simulink model "X5_PathTesting"  (R2024b)
settings: Solver=VariableStepAuto  StartTime=0.0  StopTime=20  RelTol=1e-3
libraries: Mako_Dynamics x3, dspinverses x2, g_block x1
(part 1 of 2)
settings Model: Creator=pinto  LastModifiedBy=pinto

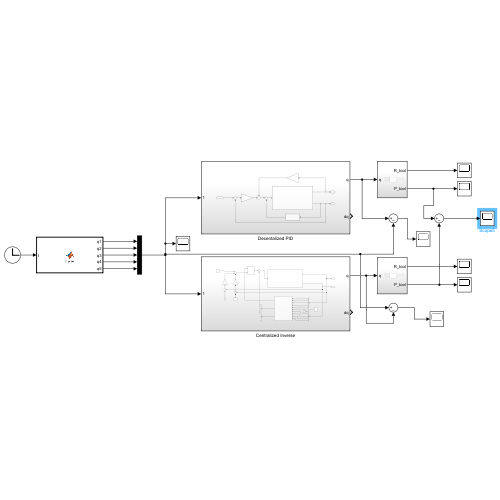
[thumbnail: Simulink's stored preview of the top-level diagram]
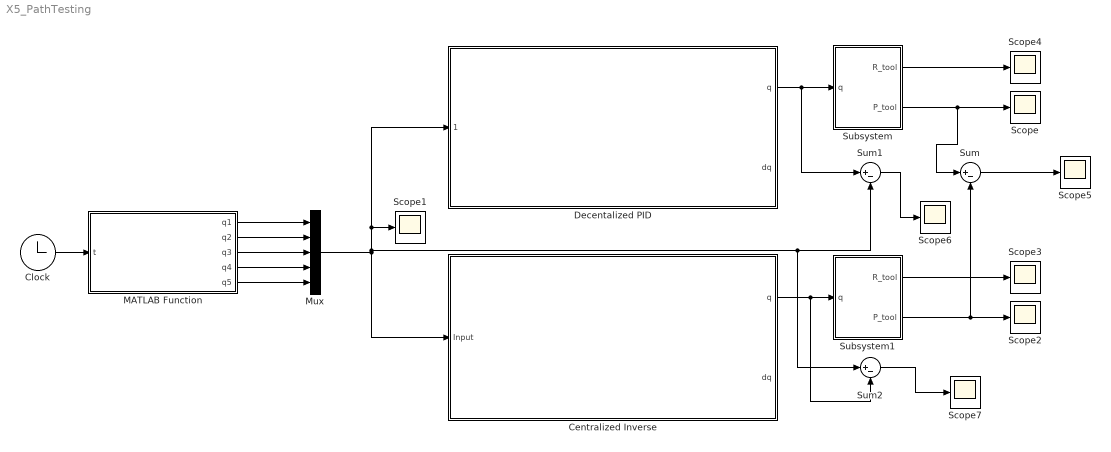
== system X5_PathTesting ==
  Centralized Inverse : Subsystem
  Clock : Clock
  Decentalized PID : Subsystem
  MATLAB Function : MATLAB Function  TreatAsAtomicUnit=on
  Mux : Mux  Inputs=5
  Scope{,1..7} (8 alike) : Scope
  Subsystem : Subsystem
  Subsystem1 : Subsystem
  Sum : Sum  Inputs=|+-
  Sum1 : Sum  Inputs=|+-
  Sum2 : Sum  Inputs=|+-
  wires:
  Clock/1 -> MATLAB Function/1(t)
  Decentalized PID/1(q) -> Sum1/1, Subsystem/1(q)
  Centralized Inverse/1(q) -> Sum2/2, Subsystem1/1(q)
  Subsystem/2(P_tool) -> Sum/1, Scope/1
  Subsystem1/2(P_tool) -> Sum/2, Scope2/1
  Subsystem1/1(R_tool) -> Scope3/1
  Subsystem/1(R_tool) -> Scope4/1
  Sum/1 -> Scope5/1
  MATLAB Function/2(q2) -> Mux/2
  Mux/1 -> Decentalized PID/1(1), Scope1/1, Sum2/1, Sum1/2, Centralized Inverse/1(Input)
  MATLAB Function/1(q1) -> Mux/1
  MATLAB Function/3(q3) -> Mux/3
  MATLAB Function/4(q4) -> Mux/4
  MATLAB Function/5(q5) -> Mux/5
  Sum1/1 -> Scope6/1
  Sum2/1 -> Scope7/1

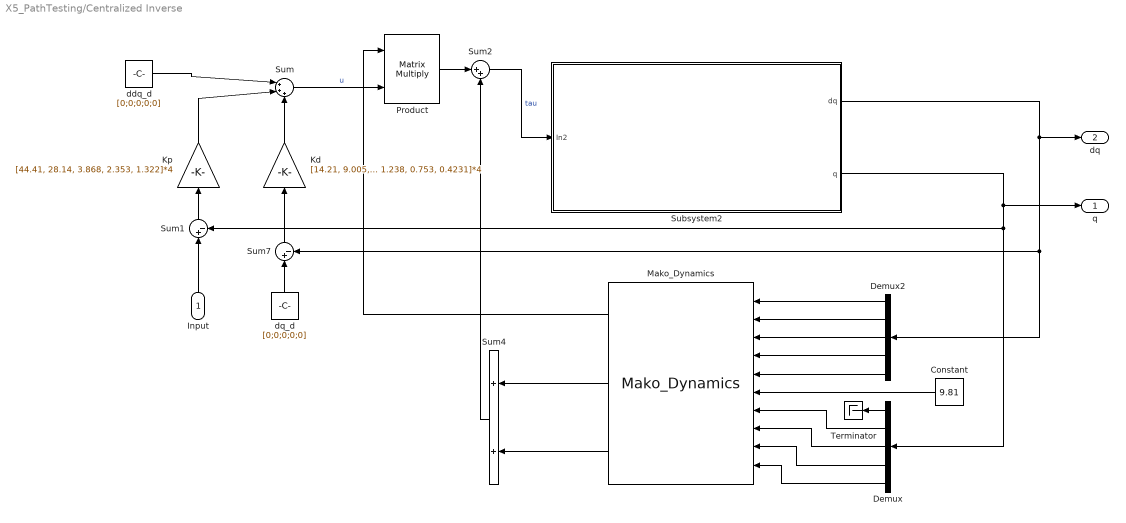
== system X5_PathTesting/Centralized Inverse ==
  Input : Inport
  Constant : Constant  Value=9.81
  Demux : Demux  Outputs=5
  Demux2 : Demux  Outputs=5
  Kd : Gain  Gain=[14.21, 9.005, 1.238, 0.753, 0.4231]*4
  Kp : Gain  Gain=[44.41, 28.14, 3.868, 2.353, 1.322]*4
  Mako_Dynamics : Mako_Dynamics/Mako_Dynamics  SystemSampleTime=-1  VariantActivationTime=update diagram  AllowFlexibleInterface=on  Latency=0  AutoFrameSizeCalculation=off
  Product : Product  Multiplication=Matrix(*)
  Subsystem2 : Subsystem
  Sum : Sum  Inputs=|+++
  Sum1 : Sum  Inputs=|+-
  Sum2 : Sum  Inputs=|++
  Sum4 : Sum
  Sum7 : Sum  Inputs=|+-
  Terminator : Terminator
  ddq_d : Constant  Value=[0;0;0;0;0]
  dq_d : Constant  Value=[0;0;0;0;0]
  q : Outport
  dq : Outport  Port=2
  wires:
  Demux/1 -> Terminator/1
  Demux2/1 -> Mako_Dynamics/1
  Kp/1 -> Sum/2
  ddq_d/1 -> Sum/1
  Product/1 -> Sum2/1
  Input/1 -> Sum1/1
  Subsystem2/2(q) -> Sum1/2, Demux/1, q/1
  Sum2/1 -> Subsystem2/1(In2)  "tau"
  Demux2/2 -> Mako_Dynamics/2
  Kd/1 -> Sum/3
  Sum1/1 -> Kp/1
  dq_d/1 -> Sum7/1
  Mako_Dynamics/1 -> Product/1
  Mako_Dynamics/3 -> Sum4/2
  Sum/1 -> Product/2  "u"
  Sum4/1 -> Sum2/2
  Demux2/3 -> Mako_Dynamics/3
  Subsystem2/1(dq) -> dq/1, Demux2/1, Sum7/2
  Sum7/1 -> Kd/1
  Demux2/5 -> Mako_Dynamics/5
  Demux2/4 -> Mako_Dynamics/4
  Mako_Dynamics/2 -> Sum4/1
  Demux/2 -> Mako_Dynamics/7
  Demux/3 -> Mako_Dynamics/8
  Demux/4 -> Mako_Dynamics/9
  Demux/5 -> Mako_Dynamics/10
  Constant/1 -> Mako_Dynamics/6

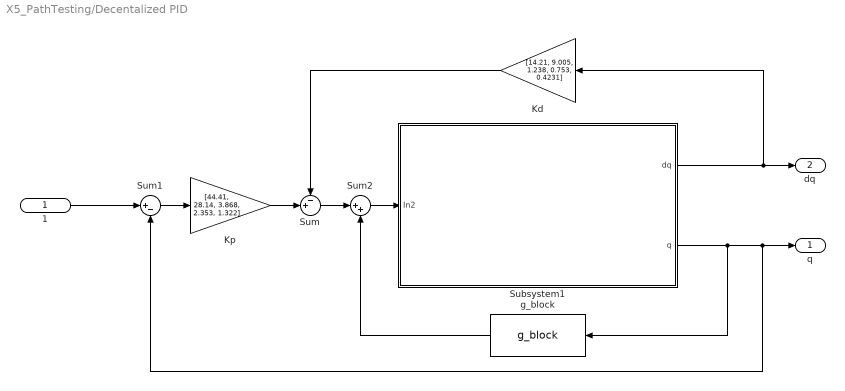
== system X5_PathTesting/Decentalized PID ==
  1 : Inport
  Kd : Gain  Gain=[14.21, 9.005, 1.238, 0.753, 0.4231]
  Kp : Gain  Gain=[44.41, 28.14, 3.868, 2.353, 1.322]
  Subsystem1 : Subsystem
  Sum : Sum  Inputs=-+|
  Sum1 : Sum  Inputs=|+-
  Sum2 : Sum  Inputs=|++
  g_block : g_block/g_block  SystemSampleTime=-1  VariantActivationTime=update diagram  AllowFlexibleInterface=on  Latency=0  AutoFrameSizeCalculation=off
  q : Outport
  dq : Outport  Port=2
  wires:
  Sum1/1 -> Kp/1
  1/1 -> Sum1/1
  Subsystem1/1(dq) -> dq/1, Kd/1
  Kd/1 -> Sum/1
  Sum2/1 -> Subsystem1/1(In2)
  Subsystem1/2(q) -> g_block/1, q/1, Sum1/2
  g_block/1 -> Sum2/2
  Kp/1 -> Sum/2
  Sum/1 -> Sum2/1

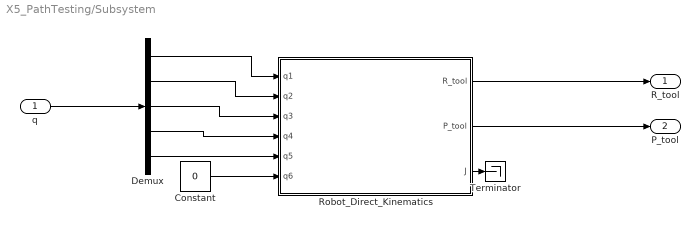
== system X5_PathTesting/Subsystem ==
  q : Inport
  Constant : Constant  Value=0
  Demux : Demux  Outputs=5
  Robot_Direct_Kinematics : MATLAB Function  TreatAsAtomicUnit=on
  Terminator : Terminator
  R_tool : Outport
  P_tool : Outport  Port=2
  wires:
  q/1 -> Demux/1
  Demux/1 -> Robot_Direct_Kinematics/1(q1)
  Demux/2 -> Robot_Direct_Kinematics/2(q2)
  Demux/3 -> Robot_Direct_Kinematics/3(q3)
  Demux/4 -> Robot_Direct_Kinematics/4(q4)
  Demux/5 -> Robot_Direct_Kinematics/5(q5)
  Constant/1 -> Robot_Direct_Kinematics/6(q6)
  Robot_Direct_Kinematics/1(R_tool) -> R_tool/1
  Robot_Direct_Kinematics/3(J) -> Terminator/1
  Robot_Direct_Kinematics/2(P_tool) -> P_tool/1

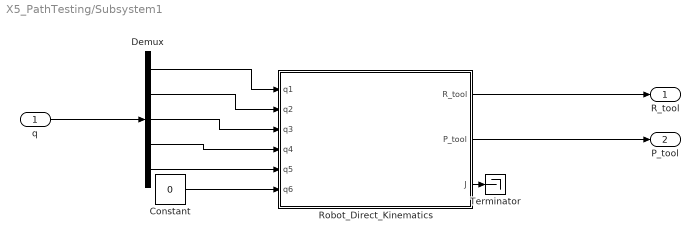
== system X5_PathTesting/Subsystem1 ==
  q : Inport
  Constant : Constant  Value=0
  Demux : Demux  Outputs=5
  Robot_Direct_Kinematics : MATLAB Function  TreatAsAtomicUnit=on
  Terminator : Terminator
  R_tool : Outport
  P_tool : Outport  Port=2
  wires:
  q/1 -> Demux/1
  Demux/1 -> Robot_Direct_Kinematics/1(q1)
  Demux/2 -> Robot_Direct_Kinematics/2(q2)
  Demux/3 -> Robot_Direct_Kinematics/3(q3)
  Demux/4 -> Robot_Direct_Kinematics/4(q4)
  Demux/5 -> Robot_Direct_Kinematics/5(q5)
  Constant/1 -> Robot_Direct_Kinematics/6(q6)
  Robot_Direct_Kinematics/1(R_tool) -> R_tool/1
  Robot_Direct_Kinematics/3(J) -> Terminator/1
  Robot_Direct_Kinematics/2(P_tool) -> P_tool/1

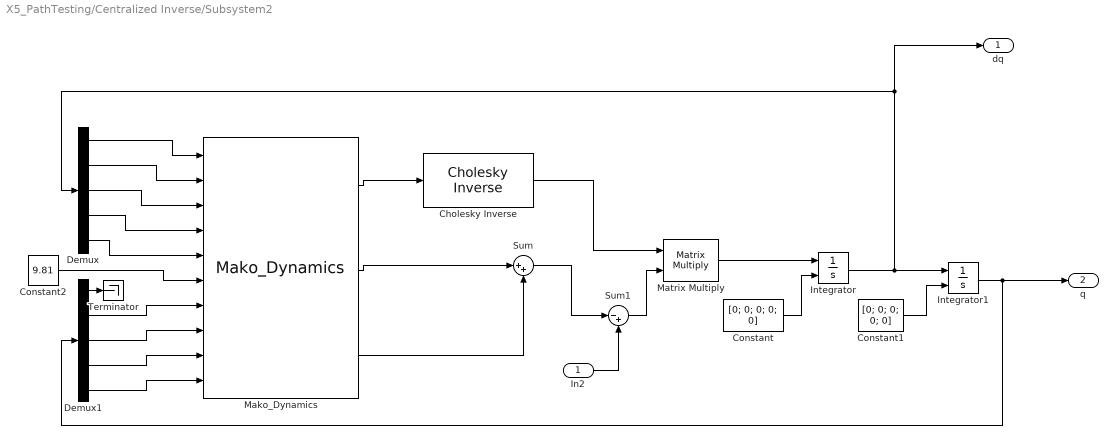
== system X5_PathTesting/Centralized Inverse/Subsystem2 ==
  In2 : Inport
  Cholesky Inverse : dspinverses/Cholesky Inverse  errmode=Warning
  Constant : Constant  Value=[0; 0; 0; 0; 0]
  Constant1 : Constant  Value=[0; 0; 0; 0; 0]
  Constant2 : Constant  Value=9.81
  Demux : Demux  Outputs=5
  Demux1 : Demux  Outputs=5
  Integrator : Integrator  InitialConditionSource=external  InitialCondition=[0.01, 0.01, 0.01]
  Integrator1 : Integrator  InitialConditionSource=external  InitialCondition=[0.01, 0.01, 0.01]
  Mako_Dynamics : Mako_Dynamics/Mako_Dynamics  SystemSampleTime=-1  VariantActivationTime=update diagram  AllowFlexibleInterface=on  Latency=0  AutoFrameSizeCalculation=off
  Matrix Multiply : Product  Multiplication=Matrix(*)
  Sum : Sum  Inputs=|++
  Sum1 : Sum  Inputs=|-+
  Terminator : Terminator
  dq : Outport
  q : Outport  Port=2
  wires:
  Sum/1 -> Sum1/1
  Demux/3 -> Mako_Dynamics/3
  Integrator/1 -> Integrator1/1, Demux/1, dq/1
  Matrix Multiply/1 -> Integrator/1
  Demux/4 -> Mako_Dynamics/4
  Demux/2 -> Mako_Dynamics/2
  Constant1/1 -> Integrator1/2
  Integrator1/1 -> q/1, Demux1/1
  Mako_Dynamics/1 -> Cholesky Inverse/1
  Cholesky Inverse/1 -> Matrix Multiply/1
  Constant/1 -> Integrator/2
  Sum1/1 -> Matrix Multiply/2
  Demux/1 -> Mako_Dynamics/1
  In2/1 -> Sum1/2
  Demux/5 -> Mako_Dynamics/5
  Mako_Dynamics/2 -> Sum/1
  Mako_Dynamics/3 -> Sum/2
  Demux1/1 -> Terminator/1
  Constant2/1 -> Mako_Dynamics/6
  Demux1/2 -> Mako_Dynamics/7
  Demux1/3 -> Mako_Dynamics/8
  Demux1/4 -> Mako_Dynamics/9
  Demux1/5 -> Mako_Dynamics/10

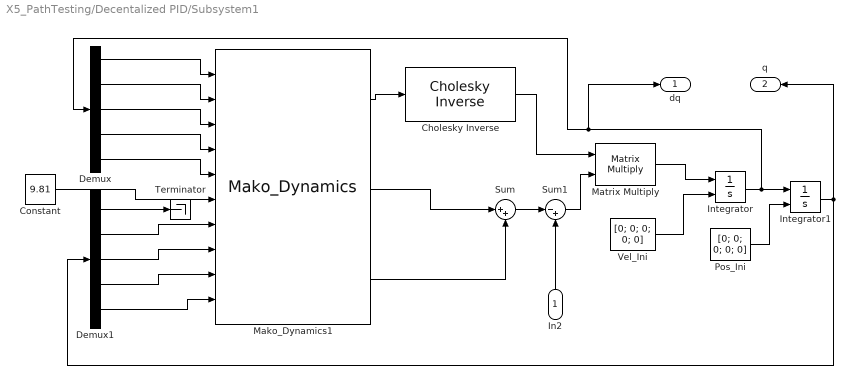
== system X5_PathTesting/Decentalized PID/Subsystem1 ==
  In2 : Inport
  Cholesky Inverse : dspinverses/Cholesky Inverse  errmode=Warning
  Constant : Constant  Value=9.81
  Demux : Demux  Outputs=5
  Demux1 : Demux  Outputs=5
  Integrator : Integrator  InitialConditionSource=external  InitialCondition=[0.01, 0.01, 0.01]
  Integrator1 : Integrator  InitialConditionSource=external  InitialCondition=[0.01, 0.01, 0.01]
  Mako_Dynamics1 : Mako_Dynamics/Mako_Dynamics  SystemSampleTime=-1  VariantActivationTime=update diagram  AllowFlexibleInterface=on  Latency=0  AutoFrameSizeCalculation=off
  Matrix Multiply : Product  Multiplication=Matrix(*)
  Pos_Ini : Constant  Value=[0; 0; 0; 0; 0]
  Sum : Sum  Inputs=|++
  Sum1 : Sum  Inputs=|-+
  Terminator : Terminator
  Vel_Ini : Constant  Value=[0; 0; 0; 0; 0]
  dq : Outport
  q : Outport  Port=2
  wires:
  Sum/1 -> Sum1/1
  Mako_Dynamics1/3 -> Sum/2
  Demux/3 -> Mako_Dynamics1/3
  Integrator/1 -> Integrator1/1, Demux/1, dq/1
  Matrix Multiply/1 -> Integrator/1
  Demux/4 -> Mako_Dynamics1/4
  Demux/2 -> Mako_Dynamics1/2
  Pos_Ini/1 -> Integrator1/2
  Integrator1/1 -> q/1, Demux1/1
  Mako_Dynamics1/1 -> Cholesky Inverse/1
  Cholesky Inverse/1 -> Matrix Multiply/1
  Vel_Ini/1 -> Integrator/2
  Sum1/1 -> Matrix Multiply/2
  Demux/1 -> Mako_Dynamics1/1
  In2/1 -> Sum1/2
  Mako_Dynamics1/2 -> Sum/1
  Demux/5 -> Mako_Dynamics1/5
  Demux1/1 -> Terminator/1
  Constant/1 -> Mako_Dynamics1/6
  Demux1/2 -> Mako_Dynamics1/7
  Demux1/3 -> Mako_Dynamics1/8
  Demux1/4 -> Mako_Dynamics1/9
  Demux1/5 -> Mako_Dynamics1/10

== matlab function X5_PathTesting/MATLAB Function ==
  data: t input; q1 output; q2 output; q3 output; q4 output; q5 output
function [q1,q2,q3,q4,q5] = Path(t)
    T = 20;
    t = min(max(t,0),T);
    s = 4*(t/T)*(1 - t/T);

    q_start = [0; 0; 0; 0; 0];
    q_peak  = [-0.4; -0.3; -0.2; 0.3; 0.3];
    q       = q_start + s*(q_peak - q_start);

    q1 = q(1);
    q2 = q(2);
    q3 = q(3);
    q4 = q(4);
    q5 = q(5);
end

== matlab function X5_PathTesting/Subsystem/Robot_Direct_Kinematics ==
  data: q1 input; R_tool output; q2 input; q3 input; q4 input; q5 input; q6 input; P_tool output; J output
function [R_tool,P_tool,J] = Robot_Direct_Kinematics(q1,q2,q3,q4,q5,q6)
%#codegen

%    This function was generated by the Symbolic Math Toolbox version 24.2.
%    24-May-2025 22:37:09

% q1 = complex(q1);  % if required to enforce complex operations
% q2 = complex(q2);  % if required to enforce complex operations
% q3 = complex(q3);  % if required to enforce complex operations
% q4 = complex(q4);  % if required to enforce complex operations
% q5 = complex(q5);  % if required to enforce complex operations
% q6 = complex(q6);  % if required to enforce complex operations
et1 = cos(q5).*sin(q1).*sin(q3).*sqrt(sqrt(2.0)+2.0).*(-1.0./2.0)-(cos(q1).*cos(q2).*sin(q4).*sin(q6).*sqrt(-sqrt(2.0)+2.0))./2.0-(cos(q3).*cos(q4).*sin(q1).*sin(q6).*sqrt(-sqrt(2.0)+2.0))./2.0-(cos(q6).*sin(q1).*sin(q3).*sin(q5).*sqrt(-sqrt(2.0)+2.0))./2.0-(cos(q1).*cos(q3).*cos(q5).*sin(q2).*sqrt(sqrt(2.0)+2.0))./2.0-(cos(q1).*cos(q2).*cos(q4).*sin(q5).*sqrt(sqrt(2.0)+2.0))./2.0+(cos(q3).*sin(q1).*sin(q4).*sin(q5).*sqrt(sqrt(2.0)+2.0))./2.0;
et2 = (cos(q1).*cos(q2).*cos(q4).*cos(q5).*cos(q6).*sqrt(-sqrt(2.0)+2.0))./2.0-(cos(q1).*cos(q3).*cos(q6).*sin(q2).*sin(q5).*sqrt(-sqrt(2.0)+2.0))./2.0-(cos(q3).*cos(q5).*cos(q6).*sin(q1).*sin(q4).*sqrt(-sqrt(2.0)+2.0))./2.0+(cos(q1).*cos(q4).*sin(q2).*sin(q3).*sin(q6).*sqrt(-sqrt(2.0)+2.0))./2.0-(cos(q1).*sin(q2).*sin(q3).*sin(q4).*sin(q5).*sqrt(sqrt(2.0)+2.0))./2.0+(cos(q1).*cos(q5).*cos(q6).*sin(q2).*sin(q3).*sin(q4).*sqrt(-sqrt(2.0)+2.0))./2.0;
et3 = cos(q1).*cos(q5).*sin(q3).*sqrt(sqrt(2.0)+2.0).*(-1.0./2.0)-(cos(q1).*cos(q3).*cos(q4).*sin(q6).*sqrt(-sqrt(2.0)+2.0))./2.0-(cos(q1).*cos(q6).*sin(q3).*sin(q5).*sqrt(-sqrt(2.0)+2.0))./2.0+(cos(q2).*sin(q1).*sin(q4).*sin(q6).*sqrt(-sqrt(2.0)+2.0))./2.0+(cos(q3).*cos(q5).*sin(q1).*sin(q2).*sqrt(sqrt(2.0)+2.0))./2.0+(cos(q2).*cos(q4).*sin(q1).*sin(q5).*sqrt(sqrt(2.0)+2.0))./2.0+(cos(q1).*cos(q3).*sin(q4).*sin(q5).*sqrt(sqrt(2.0)+2.0))./2.0-(cos(q2).*cos(q4).*cos(q5).*cos(q6).*sin(q1).*sqrt(-sqrt(2.0)+2.0))./2.0;
et4 = cos(q1).*cos(q3).*cos(q5).*cos(q6).*sin(q4).*sqrt(-sqrt(2.0)+2.0).*(-1.0./2.0)+(cos(q3).*cos(q6).*sin(q1).*sin(q2).*sin(q5).*sqrt(-sqrt(2.0)+2.0))./2.0-(cos(q4).*sin(q1).*sin(q2).*sin(q3).*sin(q6).*sqrt(-sqrt(2.0)+2.0))./2.0+(sin(q1).*sin(q2).*sin(q3).*sin(q4).*sin(q5).*sqrt(sqrt(2.0)+2.0))./2.0-(cos(q5).*cos(q6).*sin(q1).*sin(q2).*sin(q3).*sin(q4).*sqrt(-sqrt(2.0)+2.0))./2.0;
et5 = cos(q5).*sin(q1).*sin(q3).*sqrt(-sqrt(2.0)+2.0).*(-1.0./2.0)-(cos(q1).*cos(q3).*cos(q5).*sin(q2).*sqrt(-sqrt(2.0)+2.0))./2.0-(cos(q1).*cos(q2).*cos(q4).*sin(q5).*sqrt(-sqrt(2.0)+2.0))./2.0+(cos(q3).*sin(q1).*sin(q4).*sin(q5).*sqrt(-sqrt(2.0)+2.0))./2.0+(cos(q1).*cos(q2).*sin(q4).*sin(q6).*sqrt(sqrt(2.0)+2.0))./2.0+(cos(q3).*cos(q4).*sin(q1).*sin(q6).*sqrt(sqrt(2.0)+2.0))./2.0+(cos(q6).*sin(q1).*sin(q3).*sin(q5).*sqrt(sqrt(2.0)+2.0))./2.0;
et6 = cos(q1).*sin(q2).*sin(q3).*sin(q4).*sin(q5).*sqrt(-sqrt(2.0)+2.0).*(-1.0./2.0)-(cos(q1).*cos(q2).*cos(q4).*cos(q5).*cos(q6).*sqrt(sqrt(2.0)+2.0))./2.0+(cos(q1).*cos(q3).*cos(q6).*sin(q2).*sin(q5).*sqrt(sqrt(2.0)+2.0))./2.0+(cos(q3).*cos(q5).*cos(q6).*sin(q1).*sin(q4).*sqrt(sqrt(2.0)+2.0))./2.0-(cos(q1).*cos(q4).*sin(q2).*sin(q3).*sin(q6).*sqrt(sqrt(2.0)+2.0))./2.0-(cos(q1).*cos(q5).*cos(q6).*sin(q2).*sin(q3).*sin(q4).*sqrt(sqrt(2.0)+2.0))./2.0;
et7 = cos(q1).*cos(q5).*sin(q3).*sqrt(-sqrt(2.0)+2.0).*(-1.0./2.0)+(cos(q3).*cos(q5).*sin(q1).*sin(q2).*sqrt(-sqrt(2.0)+2.0))./2.0+(cos(q2).*cos(q4).*sin(q1).*sin(q5).*sqrt(-sqrt(2.0)+2.0))./2.0+(cos(q1).*cos(q3).*sin(q4).*sin(q5).*sqrt(-sqrt(2.0)+2.0))./2.0+(cos(q1).*cos(q3).*cos(q4).*sin(q6).*sqrt(sqrt(2.0)+2.0))./2.0+(cos(q1).*cos(q6).*sin(q3).*sin(q5).*sqrt(sqrt(2.0)+2.0))./2.0-(cos(q2).*sin(q1).*sin(q4).*sin(q6).*sqrt(sqrt(2.0)+2.0))./2.0;
et8 = (sin(q1).*sin(q2).*sin(q3).*sin(q4).*sin(q5).*sqrt(-sqrt(2.0)+2.0))./2.0+(cos(q2).*cos(q4).*cos(q5).*cos(q6).*sin(q1).*sqrt(sqrt(2.0)+2.0))./2.0+(cos(q1).*cos(q3).*cos(q5).*cos(q6).*sin(q4).*sqrt(sqrt(2.0)+2.0))./2.0-(cos(q3).*cos(q6).*sin(q1).*sin(q2).*sin(q5).*sqrt(sqrt(2.0)+2.0))./2.0+(cos(q4).*sin(q1).*sin(q2).*sin(q3).*sin(q6).*sqrt(sqrt(2.0)+2.0))./2.0+(cos(q5).*cos(q6).*sin(q1).*sin(q2).*sin(q3).*sin(q4).*sqrt(sqrt(2.0)+2.0))./2.0;
mt1 = [cos(q1).*cos(q3).*cos(q4).*cos(q6)-cos(q2).*cos(q6).*sin(q1).*sin(q4)-cos(q1).*sin(q3).*sin(q5).*sin(q6)-cos(q2).*cos(q4).*cos(q5).*sin(q1).*sin(q6)-cos(q1).*cos(q3).*cos(q5).*sin(q4).*sin(q6)+cos(q4).*cos(q6).*sin(q1).*sin(q2).*sin(q3)+cos(q3).*sin(q1).*sin(q2).*sin(q5).*sin(q6)-cos(q5).*sin(q1).*sin(q2).*sin(q3).*sin(q4).*sin(q6),cos(q1).*cos(q2).*cos(q6).*sin(q4)+cos(q3).*cos(q4).*cos(q6).*sin(q1)-sin(q1).*sin(q3).*sin(q5).*sin(q6)+cos(q1).*cos(q2).*cos(q4).*cos(q5).*sin(q6)-cos(q1).*cos(q4).*cos(q6).*sin(q2).*sin(q3)-cos(q1).*cos(q3).*sin(q2).*sin(q5).*sin(q6)-cos(q3).*cos(q5).*sin(q1).*sin(q4).*sin(q6)+cos(q1).*cos(q5).*sin(q2).*sin(q3).*sin(q4).*sin(q6)];
mt2 = [cos(q6).*sin(q2).*sin(q4)+cos(q2).*cos(q4).*cos(q6).*sin(q3)+cos(q2).*cos(q3).*sin(q5).*sin(q6)+cos(q4).*cos(q5).*sin(q2).*sin(q6)-cos(q2).*cos(q5).*sin(q3).*sin(q4).*sin(q6),et3+et4,et1+et2];
mt3 = [cos(q4).*sin(q2).*sin(q5).*sqrt(sqrt(2.0)+2.0).*(-1.0./2.0)-(sin(q2).*sin(q4).*sin(q6).*sqrt(-sqrt(2.0)+2.0))./2.0+(cos(q2).*cos(q3).*cos(q5).*sqrt(sqrt(2.0)+2.0))./2.0+(cos(q2).*cos(q3).*cos(q6).*sin(q5).*sqrt(-sqrt(2.0)+2.0))./2.0+(cos(q4).*cos(q5).*cos(q6).*sin(q2).*sqrt(-sqrt(2.0)+2.0))./2.0-(cos(q2).*cos(q4).*sin(q3).*sin(q6).*sqrt(-sqrt(2.0)+2.0))./2.0+(cos(q2).*sin(q3).*sin(q4).*sin(q5).*sqrt(sqrt(2.0)+2.0))./2.0-(cos(q2).*cos(q5).*cos(q6).*sin(q3).*sin(q4).*sqrt(-sqrt(2.0)+2.0))./2.0];
mt4 = [et7+et8,et5+et6,(sin(q2).*sin(q4).*sin(q6).*sqrt(sqrt(2.0)+2.0))./2.0+(cos(q2).*cos(q3).*cos(q5).*sqrt(-sqrt(2.0)+2.0))./2.0-(cos(q4).*sin(q2).*sin(q5).*sqrt(-sqrt(2.0)+2.0))./2.0+(cos(q2).*sin(q3).*sin(q4).*sin(q5).*sqrt(-sqrt(2.0)+2.0))./2.0-(cos(q2).*cos(q3).*cos(q6).*sin(q5).*sqrt(sqrt(2.0)+2.0))./2.0-(cos(q4).*cos(q5).*cos(q6).*sin(q2).*sqrt(sqrt(2.0)+2.0))./2.0+(cos(q2).*cos(q4).*sin(q3).*sin(q6).*sqrt(sqrt(2.0)+2.0))./2.0+(cos(q2).*cos(q5).*cos(q6).*sin(q3).*sin(q4).*sqrt(sqrt(2.0)+2.0))./2.0];
R_tool = reshape([mt1,mt2,mt3,mt4],3,3);
if nargout > 1
    et9 = sin(q2).*(2.0./5.0)+(cos(q4).*sin(q2))./1.0e+1+(sin(q2).*sin(q4))./2.0-(cos(q2).*cos(q3).*cos(q5))./1.0e+1+(cos(q2).*cos(q4).*sin(q3))./2.0-(cos(q2).*sin(q3).*sin(q4))./1.0e+1+(cos(q4).*sin(q2).*sin(q5))./1.0e+1+sin(q2).*sin(q4).*sin(q6).*sqrt(sqrt(2.0)+2.0).*(3.0./4.0e+1)+cos(q2).*cos(q3).*cos(q5).*sqrt(-sqrt(2.0)+2.0).*(3.0./4.0e+1)-cos(q4).*sin(q2).*sin(q5).*sqrt(-sqrt(2.0)+2.0).*(3.0./4.0e+1)-(cos(q2).*sin(q3).*sin(q4).*sin(q5))./1.0e+1+cos(q2).*sin(q3).*sin(q4).*sin(q5).*sqrt(-sqrt(2.0)+2.0).*(3.0./4.0e+1);
    et10 = cos(q2).*cos(q3).*cos(q6).*sin(q5).*sqrt(sqrt(2.0)+2.0).*(-3.0./4.0e+1)-cos(q4).*cos(q5).*cos(q6).*sin(q2).*sqrt(sqrt(2.0)+2.0).*(3.0./4.0e+1)+cos(q2).*cos(q4).*sin(q3).*sin(q6).*sqrt(sqrt(2.0)+2.0).*(3.0./4.0e+1)+cos(q2).*cos(q5).*cos(q6).*sin(q3).*sin(q4).*sqrt(sqrt(2.0)+2.0).*(3.0./4.0e+1);
    et11 = cos(q1).*cos(q2).*(2.0./5.0)+(cos(q1).*cos(q2).*cos(q4))./1.0e+1+(cos(q1).*cos(q2).*sin(q4))./2.0+(cos(q3).*cos(q4).*sin(q1))./2.0-(cos(q3).*sin(q1).*sin(q4))./1.0e+1+(cos(q5).*sin(q1).*sin(q3))./1.0e+1-cos(q5).*sin(q1).*sin(q3).*sqrt(-sqrt(2.0)+2.0).*(3.0./4.0e+1)+(cos(q1).*cos(q3).*cos(q5).*sin(q2))./1.0e+1+(cos(q1).*cos(q2).*cos(q4).*sin(q5))./1.0e+1-(cos(q1).*cos(q4).*sin(q2).*sin(q3))./2.0+(cos(q1).*sin(q2).*sin(q3).*sin(q4))./1.0e+1-(cos(q3).*sin(q1).*sin(q4).*sin(q5))./1.0e+1-cos(q1).*cos(q3).*cos(q5).*sin(q2).*sqrt(-sqrt(2.0)+2.0).*(3.0./4.0e+1);
    et12 = cos(q1).*cos(q2).*cos(q4).*sin(q5).*sqrt(-sqrt(2.0)+2.0).*(-3.0./4.0e+1)+cos(q3).*sin(q1).*sin(q4).*sin(q5).*sqrt(-sqrt(2.0)+2.0).*(3.0./4.0e+1)+(cos(q1).*sin(q2).*sin(q3).*sin(q4).*sin(q5))./1.0e+1+cos(q1).*cos(q2).*sin(q4).*sin(q6).*sqrt(sqrt(2.0)+2.0).*(3.0./4.0e+1)+cos(q3).*cos(q4).*sin(q1).*sin(q6).*sqrt(sqrt(2.0)+2.0).*(3.0./4.0e+1)+cos(q6).*sin(q1).*sin(q3).*sin(q5).*sqrt(sqrt(2.0)+2.0).*(3.0./4.0e+1)-cos(q1).*sin(q2).*sin(q3).*sin(q4).*sin(q5).*sqrt(-sqrt(2.0)+2.0).*(3.0./4.0e+1)-cos(q1).*cos(q2).*cos(q4).*cos(q5).*cos(q6).*sqrt(sqrt(2.0)+2.0).*(3.0./4.0e+1);
    et13 = cos(q1).*cos(q3).*cos(q6).*sin(q2).*sin(q5).*sqrt(sqrt(2.0)+2.0).*(3.0./4.0e+1)+cos(q3).*cos(q5).*cos(q6).*sin(q1).*sin(q4).*sqrt(sqrt(2.0)+2.0).*(3.0./4.0e+1)-cos(q1).*cos(q4).*sin(q2).*sin(q3).*sin(q6).*sqrt(sqrt(2.0)+2.0).*(3.0./4.0e+1)-cos(q1).*cos(q5).*cos(q6).*sin(q2).*sin(q3).*sin(q4).*sqrt(sqrt(2.0)+2.0).*(3.0./4.0e+1);
    et14 = cos(q2).*sin(q1).*(-2.0./5.0)+(cos(q1).*cos(q3).*cos(q4))./2.0-(cos(q2).*cos(q4).*sin(q1))./1.0e+1-(cos(q1).*cos(q3).*sin(q4))./1.0e+1+(cos(q1).*cos(q5).*sin(q3))./1.0e+1-(cos(q2).*sin(q1).*sin(q4))./2.0-cos(q1).*cos(q5).*sin(q3).*sqrt(-sqrt(2.0)+2.0).*(3.0./4.0e+1)-(cos(q3).*cos(q5).*sin(q1).*sin(q2))./1.0e+1-(cos(q2).*cos(q4).*sin(q1).*sin(q5))./1.0e+1-(cos(q1).*cos(q3).*sin(q4).*sin(q5))./1.0e+1+(cos(q4).*sin(q1).*sin(q2).*sin(q3))./2.0-(sin(q1).*sin(q2).*sin(q3).*sin(q4))./1.0e+1+cos(q3).*cos(q5).*sin(q1).*sin(q2).*sqrt(-sqrt(2.0)+2.0).*(3.0./4.0e+1);
    et15 = cos(q2).*cos(q4).*sin(q1).*sin(q5).*sqrt(-sqrt(2.0)+2.0).*(3.0./4.0e+1)+cos(q1).*cos(q3).*sin(q4).*sin(q5).*sqrt(-sqrt(2.0)+2.0).*(3.0./4.0e+1)-(sin(q1).*sin(q2).*sin(q3).*sin(q4).*sin(q5))./1.0e+1+cos(q1).*cos(q3).*cos(q4).*sin(q6).*sqrt(sqrt(2.0)+2.0).*(3.0./4.0e+1)+cos(q1).*cos(q6).*sin(q3).*sin(q5).*sqrt(sqrt(2.0)+2.0).*(3.0./4.0e+1)-cos(q2).*sin(q1).*sin(q4).*sin(q6).*sqrt(sqrt(2.0)+2.0).*(3.0./4.0e+1)+sin(q1).*sin(q2).*sin(q3).*sin(q4).*sin(q5).*sqrt(-sqrt(2.0)+2.0).*(3.0./4.0e+1)+cos(q2).*cos(q4).*cos(q5).*cos(q6).*sin(q1).*sqrt(sqrt(2.0)+2.0).*(3.0./4.0e+1);
    et16 = cos(q1).*cos(q3).*cos(q5).*cos(q6).*sin(q4).*sqrt(sqrt(2.0)+2.0).*(3.0./4.0e+1)-cos(q3).*cos(q6).*sin(q1).*sin(q2).*sin(q5).*sqrt(sqrt(2.0)+2.0).*(3.0./4.0e+1)+cos(q4).*sin(q1).*sin(q2).*sin(q3).*sin(q6).*sqrt(sqrt(2.0)+2.0).*(3.0./4.0e+1)+cos(q5).*cos(q6).*sin(q1).*sin(q2).*sin(q3).*sin(q4).*sqrt(sqrt(2.0)+2.0).*(3.0./4.0e+1);
    P_tool = [et14+et15+et16;et11+et12+et13;et9+et10];
end
if nargout > 2
    et17 = cos(q2).*sin(q1).*(-2.0./5.0)+(cos(q1).*cos(q3).*cos(q4))./2.0-(cos(q2).*cos(q4).*sin(q1))./1.0e+1-(cos(q1).*cos(q3).*sin(q4))./1.0e+1+(cos(q1).*cos(q5).*sin(q3))./1.0e+1-(cos(q2).*sin(q1).*sin(q4))./2.0-cos(q1).*cos(q5).*sin(q3).*sqrt(-sqrt(2.0)+2.0).*(3.0./4.0e+1)-(cos(q3).*cos(q5).*sin(q1).*sin(q2))./1.0e+1-(cos(q2).*cos(q4).*sin(q1).*sin(q5))./1.0e+1-(cos(q1).*cos(q3).*sin(q4).*sin(q5))./1.0e+1+(cos(q4).*sin(q1).*sin(q2).*sin(q3))./2.0-(sin(q1).*sin(q2).*sin(q3).*sin(q4))./1.0e+1+cos(q3).*cos(q5).*sin(q1).*sin(q2).*sqrt(-sqrt(2.0)+2.0).*(3.0./4.0e+1);
    et18 = cos(q2).*cos(q4).*sin(q1).*sin(q5).*sqrt(-sqrt(2.0)+2.0).*(3.0./4.0e+1)+cos(q1).*cos(q3).*sin(q4).*sin(q5).*sqrt(-sqrt(2.0)+2.0).*(3.0./4.0e+1)-(sin(q1).*sin(q2).*sin(q3).*sin(q4).*sin(q5))./1.0e+1+cos(q1).*cos(q3).*cos(q4).*sin(q6).*sqrt(sqrt(2.0)+2.0).*(3.0./4.0e+1)+cos(q1).*cos(q6).*sin(q3).*sin(q5).*sqrt(sqrt(2.0)+2.0).*(3.0./4.0e+1)-cos(q2).*sin(q1).*sin(q4).*sin(q6).*sqrt(sqrt(2.0)+2.0).*(3.0./4.0e+1)+sin(q1).*sin(q2).*sin(q3).*sin(q4).*sin(q5).*sqrt(-sqrt(2.0)+2.0).*(3.0./4.0e+1)+cos(q2).*cos(q4).*cos(q5).*cos(q6).*sin(q1).*sqrt(sqrt(2.0)+2.0).*(3.0./4.0e+1);
    et19 = cos(q1).*cos(q3).*cos(q5).*cos(q6).*sin(q4).*sqrt(sqrt(2.0)+2.0).*(3.0./4.0e+1)-cos(q3).*cos(q6).*sin(q1).*sin(q2).*sin(q5).*sqrt(sqrt(2.0)+2.0).*(3.0./4.0e+1)+cos(q4).*sin(q1).*sin(q2).*sin(q3).*sin(q6).*sqrt(sqrt(2.0)+2.0).*(3.0./4.0e+1)+cos(q5).*cos(q6).*sin(q1).*sin(q2).*sin(q3).*sin(q4).*sqrt(sqrt(2.0)+2.0).*(3.0./4.0e+1);
    et20 = cos(q1).*cos(q2).*(-2.0./5.0)-(cos(q1).*cos(q2).*cos(q4))./1.0e+1-(cos(q1).*cos(q2).*sin(q4))./2.0-(cos(q3).*cos(q4).*sin(q1))./2.0+(cos(q3).*sin(q1).*sin(q4))./1.0e+1-(cos(q5).*sin(q1).*sin(q3))./1.0e+1+cos(q5).*sin(q1).*sin(q3).*sqrt(-sqrt(2.0)+2.0).*(3.0./4.0e+1)-(cos(q1).*cos(q3).*cos(q5).*sin(q2))./1.0e+1-(cos(q1).*cos(q2).*cos(q4).*sin(q5))./1.0e+1+(cos(q1).*cos(q4).*sin(q2).*sin(q3))./2.0-(cos(q1).*sin(q2).*sin(q3).*sin(q4))./1.0e+1+(cos(q3).*sin(q1).*sin(q4).*sin(q5))./1.0e+1+cos(q1).*cos(q3).*cos(q5).*sin(q2).*sqrt(-sqrt(2.0)+2.0).*(3.0./4.0e+1);
    et21 = cos(q1).*cos(q2).*cos(q4).*sin(q5).*sqrt(-sqrt(2.0)+2.0).*(3.0./4.0e+1)-cos(q3).*sin(q1).*sin(q4).*sin(q5).*sqrt(-sqrt(2.0)+2.0).*(3.0./4.0e+1)-(cos(q1).*sin(q2).*sin(q3).*sin(q4).*sin(q5))./1.0e+1-cos(q1).*cos(q2).*sin(q4).*sin(q6).*sqrt(sqrt(2.0)+2.0).*(3.0./4.0e+1)-cos(q3).*cos(q4).*sin(q1).*sin(q6).*sqrt(sqrt(2.0)+2.0).*(3.0./4.0e+1)-cos(q6).*sin(q1).*sin(q3).*sin(q5).*sqrt(sqrt(2.0)+2.0).*(3.0./4.0e+1)+cos(q1).*sin(q2).*sin(q3).*sin(q4).*sin(q5).*sqrt(-sqrt(2.0)+2.0).*(3.0./4.0e+1);
    et22 = cos(q1).*cos(q2).*cos(q4).*cos(q5).*cos(q6).*sqrt(sqrt(2.0)+2.0).*(3.0./4.0e+1)-cos(q1).*cos(q3).*cos(q6).*sin(q2).*sin(q5).*sqrt(sqrt(2.0)+2.0).*(3.0./4.0e+1)-cos(q3).*cos(q5).*cos(q6).*sin(q1).*sin(q4).*sqrt(sqrt(2.0)+2.0).*(3.0./4.0e+1)+cos(q1).*cos(q4).*sin(q2).*sin(q3).*sin(q6).*sqrt(sqrt(2.0)+2.0).*(3.0./4.0e+1)+cos(q1).*cos(q5).*cos(q6).*sin(q2).*sin(q3).*sin(q4).*sqrt(sqrt(2.0)+2.0).*(3.0./4.0e+1);
    et23 = cos(q2).*(2.0./5.0)+(cos(q2).*cos(q4))./1.0e+1+(cos(q2).*sin(q4))./2.0+(sin(q2).*sin(q3).*sin(q4))./1.0e+1+(cos(q3).*cos(q5).*sin(q2))./1.0e+1+(cos(q2).*cos(q4).*sin(q5))./1.0e+1-(cos(q4).*sin(q2).*sin(q3))./2.0+cos(q2).*sin(q4).*sin(q6).*sqrt(sqrt(2.0)+2.0).*(3.0./4.0e+1)-cos(q3).*cos(q5).*sin(q2).*sqrt(-sqrt(2.0)+2.0).*(3.0./4.0e+1)-cos(q2).*cos(q4).*sin(q5).*sqrt(-sqrt(2.0)+2.0).*(3.0./4.0e+1)+(sin(q2).*sin(q3).*sin(q4).*sin(q5))./1.0e+1-sin(q2).*sin(q3).*sin(q4).*sin(q5).*sqrt(-sqrt(2.0)+2.0).*(3.0./4.0e+1);
    et24 = cos(q2).*cos(q4).*cos(q5).*cos(q6).*sqrt(sqrt(2.0)+2.0).*(-3.0./4.0e+1)+cos(q3).*cos(q6).*sin(q2).*sin(q5).*sqrt(sqrt(2.0)+2.0).*(3.0./4.0e+1)-cos(q4).*sin(q2).*sin(q3).*sin(q6).*sqrt(sqrt(2.0)+2.0).*(3.0./4.0e+1)-cos(q5).*cos(q6).*sin(q2).*sin(q3).*sin(q4).*sqrt(sqrt(2.0)+2.0).*(3.0./4.0e+1);
    et25 = sin(q2).*(2.0./5.0)+(cos(q4).*sin(q2))./1.0e+1+(sin(q2).*sin(q4))./2.0-(cos(q2).*cos(q3).*cos(q5))./1.0e+1+(cos(q2).*cos(q4).*sin(q3))./2.0-(cos(q2).*sin(q3).*sin(q4))./1.0e+1+(cos(q4).*sin(q2).*sin(q5))./1.0e+1+sin(q2).*sin(q4).*sin(q6).*sqrt(sqrt(2.0)+2.0).*(3.0./4.0e+1)+cos(q2).*cos(q3).*cos(q5).*sqrt(-sqrt(2.0)+2.0).*(3.0./4.0e+1)-cos(q4).*sin(q2).*sin(q5).*sqrt(-sqrt(2.0)+2.0).*(3.0./4.0e+1)-(cos(q2).*sin(q3).*sin(q4).*sin(q5))./1.0e+1+cos(q2).*sin(q3).*sin(q4).*sin(q5).*sqrt(-sqrt(2.0)+2.0).*(3.0./4.0e+1);
    et26 = cos(q2).*cos(q3).*cos(q6).*sin(q5).*sqrt(sqrt(2.0)+2.0).*(-3.0./4.0e+1)-cos(q4).*cos(q5).*cos(q6).*sin(q2).*sqrt(sqrt(2.0)+2.0).*(3.0./4.0e+1)+cos(q2).*cos(q4).*sin(q3).*sin(q6).*sqrt(sqrt(2.0)+2.0).*(3.0./4.0e+1)+cos(q2).*cos(q5).*cos(q6).*sin(q3).*sin(q4).*sqrt(sqrt(2.0)+2.0).*(3.0./4.0e+1);
    et27 = sin(q2).*(2.0./5.0)+(cos(q4).*sin(q2))./1.0e+1+(sin(q2).*sin(q4))./2.0-(cos(q2).*cos(q3).*cos(q5))./1.0e+1+(cos(q2).*cos(q4).*sin(q3))./2.0-(cos(q2).*sin(q3).*sin(q4))./1.0e+1+(cos(q4).*sin(q2).*sin(q5))./1.0e+1+sin(q2).*sin(q4).*sin(q6).*sqrt(sqrt(2.0)+2.0).*(3.0./4.0e+1)+cos(q2).*cos(q3).*cos(q5).*sqrt(-sqrt(2.0)+2.0).*(3.0./4.0e+1)-cos(q4).*sin(q2).*sin(q5).*sqrt(-sqrt(2.0)+2.0).*(3.0./4.0e+1)-(cos(q2).*sin(q3).*sin(q4).*sin(q5))./1.0e+1+cos(q2).*sin(q3).*sin(q4).*sin(q5).*sqrt(-sqrt(2.0)+2.0).*(3.0./4.0e+1);
    et28 = cos(q2).*cos(q3).*cos(q6).*sin(q5).*sqrt(sqrt(2.0)+2.0).*(-3.0./4.0e+1)-cos(q4).*cos(q5).*cos(q6).*sin(q2).*sqrt(sqrt(2.0)+2.0).*(3.0./4.0e+1)+cos(q2).*cos(q4).*sin(q3).*sin(q6).*sqrt(sqrt(2.0)+2.0).*(3.0./4.0e+1)+cos(q2).*cos(q5).*cos(q6).*sin(q3).*sin(q4).*sqrt(sqrt(2.0)+2.0).*(3.0./4.0e+1);
    et29 = (sin(q1).*sin(q3).*sin(q4))./1.0e+1+(cos(q3).*cos(q5).*sin(q1))./1.0e+1-(cos(q4).*sin(q1).*sin(q3))./2.0-cos(q3).*cos(q5).*sin(q1).*sqrt(-sqrt(2.0)+2.0).*(3.0./4.0e+1)-(cos(q1).*cos(q3).*cos(q4).*sin(q2))./2.0+(cos(q1).*cos(q3).*sin(q2).*sin(q4))./1.0e+1-(cos(q1).*cos(q5).*sin(q2).*sin(q3))./1.0e+1+(sin(q1).*sin(q3).*sin(q4).*sin(q5))./1.0e+1+cos(q1).*cos(q5).*sin(q2).*sin(q3).*sqrt(-sqrt(2.0)+2.0).*(3.0./4.0e+1)-sin(q1).*sin(q3).*sin(q4).*sin(q5).*sqrt(-sqrt(2.0)+2.0).*(3.0./4.0e+1)+(cos(q1).*cos(q3).*sin(q2).*sin(q4).*sin(q5))./1.0e+1;
    et30 = cos(q3).*cos(q6).*sin(q1).*sin(q5).*sqrt(sqrt(2.0)+2.0).*(3.0./4.0e+1)-cos(q4).*sin(q1).*sin(q3).*sin(q6).*sqrt(sqrt(2.0)+2.0).*(3.0./4.0e+1)-cos(q1).*cos(q3).*sin(q2).*sin(q4).*sin(q5).*sqrt(-sqrt(2.0)+2.0).*(3.0./4.0e+1)-cos(q1).*cos(q3).*cos(q4).*sin(q2).*sin(q6).*sqrt(sqrt(2.0)+2.0).*(3.0./4.0e+1)-cos(q1).*cos(q6).*sin(q2).*sin(q3).*sin(q5).*sqrt(sqrt(2.0)+2.0).*(3.0./4.0e+1)-cos(q5).*cos(q6).*sin(q1).*sin(q3).*sin(q4).*sqrt(sqrt(2.0)+2.0).*(3.0./4.0e+1)-cos(q1).*cos(q3).*cos(q5).*cos(q6).*sin(q2).*sin(q4).*sqrt(sqrt(2.0)+2.0).*(3.0./4.0e+1);
    et31 = (cos(q1).*cos(q3).*cos(q5))./1.0e+1-(cos(q1).*cos(q4).*sin(q3))./2.0+(cos(q1).*sin(q3).*sin(q4))./1.0e+1-cos(q1).*cos(q3).*cos(q5).*sqrt(-sqrt(2.0)+2.0).*(3.0./4.0e+1)+(cos(q3).*cos(q4).*sin(q1).*sin(q2))./2.0-(cos(q3).*sin(q1).*sin(q2).*sin(q4))./1.0e+1+(cos(q5).*sin(q1).*sin(q2).*sin(q3))./1.0e+1+(cos(q1).*sin(q3).*sin(q4).*sin(q5))./1.0e+1-cos(q5).*sin(q1).*sin(q2).*sin(q3).*sqrt(-sqrt(2.0)+2.0).*(3.0./4.0e+1)-cos(q1).*sin(q3).*sin(q4).*sin(q5).*sqrt(-sqrt(2.0)+2.0).*(3.0./4.0e+1)-(cos(q3).*sin(q1).*sin(q2).*sin(q4).*sin(q5))./1.0e+1;
    et32 = cos(q1).*cos(q3).*cos(q6).*sin(q5).*sqrt(sqrt(2.0)+2.0).*(3.0./4.0e+1)-cos(q1).*cos(q4).*sin(q3).*sin(q6).*sqrt(sqrt(2.0)+2.0).*(3.0./4.0e+1)+cos(q3).*sin(q1).*sin(q2).*sin(q4).*sin(q5).*sqrt(-sqrt(2.0)+2.0).*(3.0./4.0e+1)-cos(q1).*cos(q5).*cos(q6).*sin(q3).*sin(q4).*sqrt(sqrt(2.0)+2.0).*(3.0./4.0e+1)+cos(q3).*cos(q4).*sin(q1).*sin(q2).*sin(q6).*sqrt(sqrt(2.0)+2.0).*(3.0./4.0e+1)+cos(q6).*sin(q1).*sin(q2).*sin(q3).*sin(q5).*sqrt(sqrt(2.0)+2.0).*(3.0./4.0e+1)+cos(q3).*cos(q5).*cos(q6).*sin(q1).*sin(q2).*sin(q4).*sqrt(sqrt(2.0)+2.0).*(3.0./4.0e+1);
    et33 = (cos(q4).*sin(q2))./2.0-(sin(q2).*sin(q4))./1.0e+1-(sin(q2).*sin(q4).*sin(q5))./1.0e+1-(cos(q2).*cos(q4).*sin(q3))./1.0e+1-(cos(q2).*sin(q3).*sin(q4))./2.0+cos(q4).*sin(q2).*sin(q6).*sqrt(sqrt(2.0)+2.0).*(3.0./4.0e+1)+sin(q2).*sin(q4).*sin(q5).*sqrt(-sqrt(2.0)+2.0).*(3.0./4.0e+1)-(cos(q2).*cos(q4).*sin(q3).*sin(q5))./1.0e+1+cos(q2).*cos(q4).*sin(q3).*sin(q5).*sqrt(-sqrt(2.0)+2.0).*(3.0./4.0e+1)+cos(q5).*cos(q6).*sin(q2).*sin(q4).*sqrt(sqrt(2.0)+2.0).*(3.0./4.0e+1)-cos(q2).*sin(q3).*sin(q4).*sin(q6).*sqrt(sqrt(2.0)+2.0).*(3.0./4.0e+1);
    et34 = cos(q2).*cos(q4).*cos(q5).*cos(q6).*sin(q3).*sqrt(sqrt(2.0)+2.0).*(3.0./4.0e+1);
    et35 = (cos(q1).*cos(q2).*cos(q4))./2.0-(cos(q1).*cos(q2).*sin(q4))./1.0e+1-(cos(q3).*cos(q4).*sin(q1))./1.0e+1-(cos(q3).*sin(q1).*sin(q4))./2.0+(cos(q1).*cos(q4).*sin(q2).*sin(q3))./1.0e+1-(cos(q1).*cos(q2).*sin(q4).*sin(q5))./1.0e+1-(cos(q3).*cos(q4).*sin(q1).*sin(q5))./1.0e+1+(cos(q1).*sin(q2).*sin(q3).*sin(q4))./2.0+cos(q1).*cos(q2).*sin(q4).*sin(q5).*sqrt(-sqrt(2.0)+2.0).*(3.0./4.0e+1)+cos(q3).*cos(q4).*sin(q1).*sin(q5).*sqrt(-sqrt(2.0)+2.0).*(3.0./4.0e+1)+(cos(q1).*cos(q4).*sin(q2).*sin(q3).*sin(q5))./1.0e+1+cos(q1).*cos(q2).*cos(q4).*sin(q6).*sqrt(sqrt(2.0)+2.0).*(3.0./4.0e+1);
    et36 = cos(q3).*sin(q1).*sin(q4).*sin(q6).*sqrt(sqrt(2.0)+2.0).*(-3.0./4.0e+1)-cos(q1).*cos(q4).*sin(q2).*sin(q3).*sin(q5).*sqrt(-sqrt(2.0)+2.0).*(3.0./4.0e+1)+cos(q1).*cos(q2).*cos(q5).*cos(q6).*sin(q4).*sqrt(sqrt(2.0)+2.0).*(3.0./4.0e+1)+cos(q3).*cos(q4).*cos(q5).*cos(q6).*sin(q1).*sqrt(sqrt(2.0)+2.0).*(3.0./4.0e+1)+cos(q1).*sin(q2).*sin(q3).*sin(q4).*sin(q6).*sqrt(sqrt(2.0)+2.0).*(3.0./4.0e+1)-cos(q1).*cos(q4).*cos(q5).*cos(q6).*sin(q2).*sin(q3).*sqrt(sqrt(2.0)+2.0).*(3.0./4.0e+1);
    et37 = cos(q1).*cos(q3).*cos(q4).*(-1.0./1.0e+1)-(cos(q2).*cos(q4).*sin(q1))./2.0-(cos(q1).*cos(q3).*sin(q4))./2.0+(cos(q2).*sin(q1).*sin(q4))./1.0e+1-(cos(q1).*cos(q3).*cos(q4).*sin(q5))./1.0e+1-(cos(q4).*sin(q1).*sin(q2).*sin(q3))./1.0e+1+(cos(q2).*sin(q1).*sin(q4).*sin(q5))./1.0e+1-(sin(q1).*sin(q2).*sin(q3).*sin(q4))./2.0+cos(q1).*cos(q3).*cos(q4).*sin(q5).*sqrt(-sqrt(2.0)+2.0).*(3.0./4.0e+1)-cos(q2).*sin(q1).*sin(q4).*sin(q5).*sqrt(-sqrt(2.0)+2.0).*(3.0./4.0e+1)-(cos(q4).*sin(q1).*sin(q2).*sin(q3).*sin(q5))./1.0e+1-cos(q2).*cos(q4).*sin(q1).*sin(q6).*sqrt(sqrt(2.0)+2.0).*(3.0./4.0e+1);
    et38 = cos(q1).*cos(q3).*sin(q4).*sin(q6).*sqrt(sqrt(2.0)+2.0).*(-3.0./4.0e+1)+cos(q4).*sin(q1).*sin(q2).*sin(q3).*sin(q5).*sqrt(-sqrt(2.0)+2.0).*(3.0./4.0e+1)+cos(q1).*cos(q3).*cos(q4).*cos(q5).*cos(q6).*sqrt(sqrt(2.0)+2.0).*(3.0./4.0e+1)-cos(q2).*cos(q5).*cos(q6).*sin(q1).*sin(q4).*sqrt(sqrt(2.0)+2.0).*(3.0./4.0e+1)-sin(q1).*sin(q2).*sin(q3).*sin(q4).*sin(q6).*sqrt(sqrt(2.0)+2.0).*(3.0./4.0e+1)+cos(q4).*cos(q5).*cos(q6).*sin(q1).*sin(q2).*sin(q3).*sqrt(sqrt(2.0)+2.0).*(3.0./4.0e+1);
    et39 = (cos(q1).*cos(q3).*cos(q4))./2.0+(cos(q1).*cos(q5).*sin(q3))./1.0e+1-(cos(q2).*sin(q1).*sin(q4))./2.0-cos(q1).*cos(q5).*sin(q3).*sqrt(-sqrt(2.0)+2.0).*(3.0./4.0e+1)-(cos(q3).*cos(q5).*sin(q1).*sin(q2))./1.0e+1-(cos(q2).*cos(q4).*sin(q1).*sin(q5))./1.0e+1-(cos(q1).*cos(q3).*sin(q4).*sin(q5))./1.0e+1+(cos(q4).*sin(q1).*sin(q2).*sin(q3))./2.0+cos(q3).*cos(q5).*sin(q1).*sin(q2).*sqrt(-sqrt(2.0)+2.0).*(3.0./4.0e+1)+cos(q2).*cos(q4).*sin(q1).*sin(q5).*sqrt(-sqrt(2.0)+2.0).*(3.0./4.0e+1)+cos(q1).*cos(q3).*sin(q4).*sin(q5).*sqrt(-sqrt(2.0)+2.0).*(3.0./4.0e+1);
    et40 = sin(q1).*sin(q2).*sin(q3).*sin(q4).*sin(q5).*(-1.0./1.0e+1)+cos(q1).*cos(q3).*cos(q4).*sin(q6).*sqrt(sqrt(2.0)+2.0).*(3.0./4.0e+1)+cos(q1).*cos(q6).*sin(q3).*sin(q5).*sqrt(sqrt(2.0)+2.0).*(3.0./4.0e+1)-cos(q2).*sin(q1).*sin(q4).*sin(q6).*sqrt(sqrt(2.0)+2.0).*(3.0./4.0e+1)+sin(q1).*sin(q2).*sin(q3).*sin(q4).*sin(q5).*sqrt(-sqrt(2.0)+2.0).*(3.0./4.0e+1)+cos(q2).*cos(q4).*cos(q5).*cos(q6).*sin(q1).*sqrt(sqrt(2.0)+2.0).*(3.0./4.0e+1)+cos(q1).*cos(q3).*cos(q5).*cos(q6).*sin(q4).*sqrt(sqrt(2.0)+2.0).*(3.0./4.0e+1)-cos(q3).*cos(q6).*sin(q1).*sin(q2).*sin(q5).*sqrt(sqrt(2.0)+2.0).*(3.0./4.0e+1);
    et41 = cos(q4).*sin(q1).*sin(q2).*sin(q3).*sin(q6).*sqrt(sqrt(2.0)+2.0).*(3.0./4.0e+1)+cos(q5).*cos(q6).*sin(q1).*sin(q2).*sin(q3).*sin(q4).*sqrt(sqrt(2.0)+2.0).*(3.0./4.0e+1);
    et42 = (sin(q2).*sin(q4))./2.0-(cos(q2).*cos(q3).*cos(q5))./1.0e+1+(cos(q2).*cos(q4).*sin(q3))./2.0+(cos(q4).*sin(q2).*sin(q5))./1.0e+1+sin(q2).*sin(q4).*sin(q6).*sqrt(sqrt(2.0)+2.0).*(3.0./4.0e+1)+cos(q2).*cos(q3).*cos(q5).*sqrt(-sqrt(2.0)+2.0).*(3.0./4.0e+1)-cos(q4).*sin(q2).*sin(q5).*sqrt(-sqrt(2.0)+2.0).*(3.0./4.0e+1)-(cos(q2).*sin(q3).*sin(q4).*sin(q5))./1.0e+1+cos(q2).*sin(q3).*sin(q4).*sin(q5).*sqrt(-sqrt(2.0)+2.0).*(3.0./4.0e+1)-cos(q2).*cos(q3).*cos(q6).*sin(q5).*sqrt(sqrt(2.0)+2.0).*(3.0./4.0e+1);
    et43 = cos(q4).*cos(q5).*cos(q6).*sin(q2).*sqrt(sqrt(2.0)+2.0).*(-3.0./4.0e+1)+cos(q2).*cos(q4).*sin(q3).*sin(q6).*sqrt(sqrt(2.0)+2.0).*(3.0./4.0e+1)+cos(q2).*cos(q5).*cos(q6).*sin(q3).*sin(q4).*sqrt(sqrt(2.0)+2.0).*(3.0./4.0e+1);
    et44 = (cos(q1).*cos(q2).*sin(q4))./2.0+(cos(q3).*cos(q4).*sin(q1))./2.0+(cos(q5).*sin(q1).*sin(q3))./1.0e+1-cos(q5).*sin(q1).*sin(q3).*sqrt(-sqrt(2.0)+2.0).*(3.0./4.0e+1)+(cos(q1).*cos(q3).*cos(q5).*sin(q2))./1.0e+1+(cos(q1).*cos(q2).*cos(q4).*sin(q5))./1.0e+1-(cos(q1).*cos(q4).*sin(q2).*sin(q3))./2.0-(cos(q3).*sin(q1).*sin(q4).*sin(q5))./1.0e+1-cos(q1).*cos(q3).*cos(q5).*sin(q2).*sqrt(-sqrt(2.0)+2.0).*(3.0./4.0e+1)-cos(q1).*cos(q2).*cos(q4).*sin(q5).*sqrt(-sqrt(2.0)+2.0).*(3.0./4.0e+1)+cos(q3).*sin(q1).*sin(q4).*sin(q5).*sqrt(-sqrt(2.0)+2.0).*(3.0./4.0e+1);
    et45 = (cos(q1).*sin(q2).*sin(q3).*sin(q4).*sin(q5))./1.0e+1+cos(q1).*cos(q2).*sin(q4).*sin(q6).*sqrt(sqrt(2.0)+2.0).*(3.0./4.0e+1)+cos(q3).*cos(q4).*sin(q1).*sin(q6).*sqrt(sqrt(2.0)+2.0).*(3.0./4.0e+1)+cos(q6).*sin(q1).*sin(q3).*sin(q5).*sqrt(sqrt(2.0)+2.0).*(3.0./4.0e+1)-cos(q1).*sin(q2).*sin(q3).*sin(q4).*sin(q5).*sqrt(-sqrt(2.0)+2.0).*(3.0./4.0e+1)-cos(q1).*cos(q2).*cos(q4).*cos(q5).*cos(q6).*sqrt(sqrt(2.0)+2.0).*(3.0./4.0e+1)+cos(q1).*cos(q3).*cos(q6).*sin(q2).*sin(q5).*sqrt(sqrt(2.0)+2.0).*(3.0./4.0e+1)+cos(q3).*cos(q5).*cos(q6).*sin(q1).*sin(q4).*sqrt(sqrt(2.0)+2.0).*(3.0./4.0e+1);
    et46 = cos(q1).*cos(q4).*sin(q2).*sin(q3).*sin(q6).*sqrt(sqrt(2.0)+2.0).*(-3.0./4.0e+1)-cos(q1).*cos(q5).*cos(q6).*sin(q2).*sin(q3).*sin(q4).*sqrt(sqrt(2.0)+2.0).*(3.0./4.0e+1);
    et47 = (sin(q2).*sin(q4))./2.0-(cos(q2).*cos(q3).*cos(q5))./1.0e+1+(cos(q2).*cos(q4).*sin(q3))./2.0+(cos(q4).*sin(q2).*sin(q5))./1.0e+1+sin(q2).*sin(q4).*sin(q6).*sqrt(sqrt(2.0)+2.0).*(3.0./4.0e+1)+cos(q2).*cos(q3).*cos(q5).*sqrt(-sqrt(2.0)+2.0).*(3.0./4.0e+1)-cos(q4).*sin(q2).*sin(q5).*sqrt(-sqrt(2.0)+2.0).*(3.0./4.0e+1)-(cos(q2).*sin(q3).*sin(q4).*sin(q5))./1.0e+1+cos(q2).*sin(q3).*sin(q4).*sin(q5).*sqrt(-sqrt(2.0)+2.0).*(3.0./4.0e+1)-cos(q2).*cos(q3).*cos(q6).*sin(q5).*sqrt(sqrt(2.0)+2.0).*(3.0./4.0e+1);
    et48 = cos(q4).*cos(q5).*cos(q6).*sin(q2).*sqrt(sqrt(2.0)+2.0).*(-3.0./4.0e+1)+cos(q2).*cos(q4).*sin(q3).*sin(q6).*sqrt(sqrt(2.0)+2.0).*(3.0./4.0e+1)+cos(q2).*cos(q5).*cos(q6).*sin(q3).*sin(q4).*sqrt(sqrt(2.0)+2.0).*(3.0./4.0e+1);
    et49 = sin(q1).*sin(q3).*sin(q5).*sin(q6).*sqrt(sqrt(2.0)+2.0).*(-3.0./4.0e+1)+cos(q1).*cos(q2).*cos(q6).*sin(q4).*sqrt(sqrt(2.0)+2.0).*(3.0./4.0e+1)+cos(q3).*cos(q4).*cos(q6).*sin(q1).*sqrt(sqrt(2.0)+2.0).*(3.0./4.0e+1)+cos(q1).*cos(q2).*cos(q4).*cos(q5).*sin(q6).*sqrt(sqrt(2.0)+2.0).*(3.0./4.0e+1)-cos(q1).*cos(q4).*cos(q6).*sin(q2).*sin(q3).*sqrt(sqrt(2.0)+2.0).*(3.0./4.0e+1)-cos(q1).*cos(q3).*sin(q2).*sin(q5).*sin(q6).*sqrt(sqrt(2.0)+2.0).*(3.0./4.0e+1)-cos(q3).*cos(q5).*sin(q1).*sin(q4).*sin(q6).*sqrt(sqrt(2.0)+2.0).*(3.0./4.0e+1);
    et50 = cos(q1).*cos(q5).*sin(q2).*sin(q3).*sin(q4).*sin(q6).*sqrt(sqrt(2.0)+2.0).*(3.0./4.0e+1);
    et51 = cos(q1).*cos(q3).*cos(q4).*cos(q6).*sqrt(sqrt(2.0)+2.0).*(3.0./4.0e+1)-cos(q2).*cos(q6).*sin(q1).*sin(q4).*sqrt(sqrt(2.0)+2.0).*(3.0./4.0e+1)-cos(q1).*sin(q3).*sin(q5).*sin(q6).*sqrt(sqrt(2.0)+2.0).*(3.0./4.0e+1)-cos(q2).*cos(q4).*cos(q5).*sin(q1).*sin(q6).*sqrt(sqrt(2.0)+2.0).*(3.0./4.0e+1)-cos(q1).*cos(q3).*cos(q5).*sin(q4).*sin(q6).*sqrt(sqrt(2.0)+2.0).*(3.0./4.0e+1)+cos(q4).*cos(q6).*sin(q1).*sin(q2).*sin(q3).*sqrt(sqrt(2.0)+2.0).*(3.0./4.0e+1)+cos(q3).*sin(q1).*sin(q2).*sin(q5).*sin(q6).*sqrt(sqrt(2.0)+2.0).*(3.0./4.0e+1);
    et52 = cos(q5).*sin(q1).*sin(q2).*sin(q3).*sin(q4).*sin(q6).*sqrt(sqrt(2.0)+2.0).*(-3.0./4.0e+1);
    mt5 = [et20+et21+et22,et17+et18+et19,0.0,0.0,0.0,1.0,sin(q1).*(et27+et28),-cos(q1).*(et25+et26),et23+et24,cos(q1),sin(q1),0.0,et31+et32,et29+et30,(cos(q2).*(cos(q3).*cos(q4).*2.0e+1-cos(q3).*sin(q4).*4.0+cos(q5).*sin(q3).*4.0-cos(q5).*sin(q3).*sqrt(-sqrt(2.0)+2.0).*3.0-cos(q3).*sin(q4).*sin(q5).*4.0+cos(q3).*cos(q4).*sin(q6).*sqrt(sqrt(2.0)+2.0).*3.0+cos(q6).*sin(q3).*sin(q5).*sqrt(sqrt(2.0)+2.0).*3.0+cos(q3).*sin(q4).*sin(q5).*sqrt(-sqrt(2.0)+2.0).*3.0+cos(q3).*cos(q5).*cos(q6).*sin(q4).*sqrt(sqrt(2.0)+2.0).*3.0))./4.0e+1,cos(q2).*sin(q1),-cos(q1).*cos(q2),-sin(q2),et37+et38];
    mt6 = [et35+et36,et33+et34,-cos(q1).*sin(q3)+cos(q3).*sin(q1).*sin(q2),-sin(q1).*sin(q3)-cos(q1).*cos(q3).*sin(q2),cos(q2).*cos(q3),-(sin(q2).*sin(q4)+cos(q2).*cos(q4).*sin(q3)).*(et44+et45+et46)+(et47+et48).*(cos(q1).*cos(q2).*sin(q4)+cos(q3).*cos(q4).*sin(q1)-cos(q1).*cos(q4).*sin(q2).*sin(q3)),(sin(q2).*sin(q4)+cos(q2).*cos(q4).*sin(q3)).*(et39+et40+et41)-(et42+et43).*(cos(q1).*cos(q3).*cos(q4)-cos(q2).*sin(q1).*sin(q4)+cos(q4).*sin(q1).*sin(q2).*sin(q3))];
    mt7 = [(cos(q2).*cos(q3).*sin(q5))./1.0e+1+(cos(q4).*cos(q5).*sin(q2))./1.0e+1-cos(q2).*cos(q3).*sin(q5).*sqrt(-sqrt(2.0)+2.0).*(3.0./4.0e+1)-cos(q4).*cos(q5).*sin(q2).*sqrt(-sqrt(2.0)+2.0).*(3.0./4.0e+1)-(cos(q2).*cos(q5).*sin(q3).*sin(q4))./1.0e+1+cos(q2).*cos(q5).*sin(q3).*sin(q4).*sqrt(-sqrt(2.0)+2.0).*(3.0./4.0e+1)-cos(q2).*cos(q3).*cos(q5).*cos(q6).*sqrt(sqrt(2.0)+2.0).*(3.0./4.0e+1)+cos(q4).*cos(q6).*sin(q2).*sin(q5).*sqrt(sqrt(2.0)+2.0).*(3.0./4.0e+1)-cos(q2).*cos(q6).*sin(q3).*sin(q4).*sin(q5).*sqrt(sqrt(2.0)+2.0).*(3.0./4.0e+1)];
    mt8 = [cos(q1).*cos(q3).*cos(q4)-cos(q2).*sin(q1).*sin(q4)+cos(q4).*sin(q1).*sin(q2).*sin(q3),cos(q1).*cos(q2).*sin(q4)+cos(q3).*cos(q4).*sin(q1)-cos(q1).*cos(q4).*sin(q2).*sin(q3),sin(q2).*sin(q4)+cos(q2).*cos(q4).*sin(q3),et51+et52,et49+et50,sqrt(sqrt(2.0)+2.0).*(cos(q6).*sin(q2).*sin(q4)+cos(q2).*cos(q4).*cos(q6).*sin(q3)+cos(q2).*cos(q3).*sin(q5).*sin(q6)+cos(q4).*cos(q5).*sin(q2).*sin(q6)-cos(q2).*cos(q5).*sin(q3).*sin(q4).*sin(q6)).*(3.0./4.0e+1),-cos(q1).*cos(q5).*sin(q3)+cos(q3).*cos(q5).*sin(q1).*sin(q2)+cos(q2).*cos(q4).*sin(q1).*sin(q5)+cos(q1).*cos(q3).*sin(q4).*sin(q5)+sin(q1).*sin(q2).*sin(q3).*sin(q4).*sin(q5)];
    mt9 = [-cos(q5).*sin(q1).*sin(q3)-cos(q1).*cos(q3).*cos(q5).*sin(q2)-cos(q1).*cos(q2).*cos(q4).*sin(q5)+cos(q3).*sin(q1).*sin(q4).*sin(q5)-cos(q1).*sin(q2).*sin(q3).*sin(q4).*sin(q5),cos(q2).*cos(q3).*cos(q5)-cos(q4).*sin(q2).*sin(q5)+cos(q2).*sin(q3).*sin(q4).*sin(q5)];
    J = reshape([mt5,mt6,mt7,mt8,mt9],6,6);
end
end
